simulink model "ADHW5p3"  (R2022b)
settings: Solver=VariableStepAuto  StartTime=0.0  StopTime=3000.0  RelTol=1e-3
libraries: vrlib x1
settings Model: Creator=izacu  LastModifiedBy=izacu

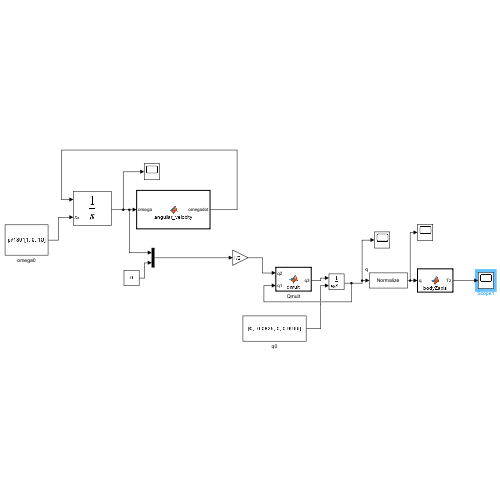
[thumbnail: Simulink's stored preview of the top-level diagram]
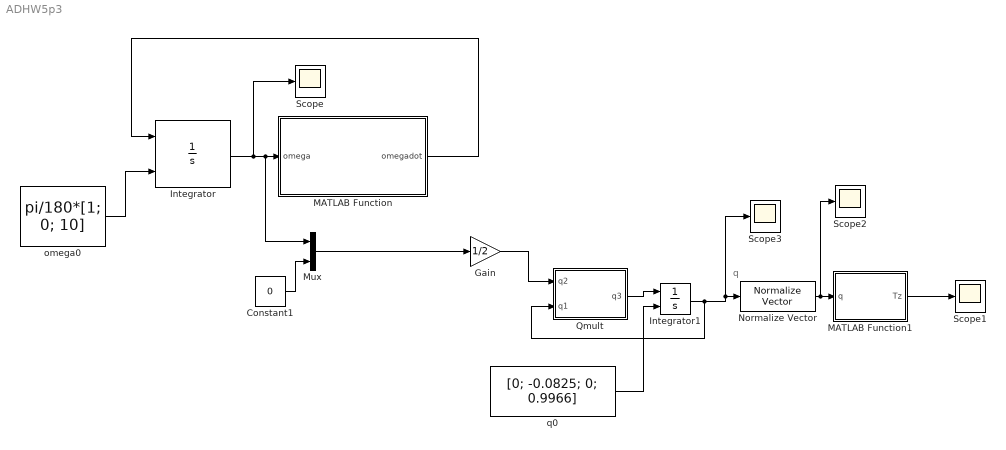
== system ADHW5p3 ==
  note: q
  Constant1 : Constant  Value=0
  Gain : Gain  Gain=1/2
  Integrator : Integrator  InitialConditionSource=external
  Integrator1 : Integrator  InitialConditionSource=external
  MATLAB Function : MATLAB Function  TreatAsAtomicUnit=on
  MATLAB Function1 : MATLAB Function  TreatAsAtomicUnit=on
  Mux : Mux  Inputs=2
  Normalize Vector : vrlib/Utilities/Normalize Vector  maxzero=0
  Qmult : MATLAB Function  TreatAsAtomicUnit=on
  Scope{,1..3} (4 alike) : Scope
  omega0 : Constant  Value=pi/180*[1; 0; 10]
  q0 : Constant  Value=[0; -0.0825; 0; 0.9966]
  wires:
  omega0/1 -> Integrator/2
  Integrator/1 -> Scope/1, Mux/1, MATLAB Function/1(omega)
  MATLAB Function/1(omegadot) -> Integrator/1
  Constant1/1 -> Mux/2
  Mux/1 -> Gain/1
  Gain/1 -> Qmult/1(q2)
  Qmult/1(q3) -> Integrator1/1
  MATLAB Function1/1(Tz) -> Scope1/1
  Integrator1/1 -> Qmult/2(q1), Scope3/1, Normalize Vector/1
  Normalize Vector/1 -> Scope2/1, MATLAB Function1/1(q)
  q0/1 -> Integrator1/2

== matlab function ADHW5p3/MATLAB Function ==
  data: omega input; omegadot output
function omegadot = angular_velocity(omega)

J = [100 0 0; 0 100 0; 0 0 60];

omegadot = -inv(J)*(cross(omega,J*omega));

== matlab function ADHW5p3/Qmult ==
  data: q2 input; q1 input; q3 output
function q3 = qmult(q2,q1)

q3 = [q2(4).*q1(1:3) + q1(4).*q2(1:3) - cross(q2(1:3),q1(1:3));
    q2(4)*q1(4) - dot(q2(1:3),q1(1:3))];

== matlab function ADHW5p3/MATLAB Function1 ==
  data: q input; Tz output
function Tz = bodyZaxis(q)
I = eye(3);
qs = q(4);

qvx = [0 -q(3) q(2); q(3) 0 -q(1); -q(2) q(1) 0];

T = I - 2*qs.*qvx + 2*qvx*qvx;

Tz = T(3,:);
